simulink subsystem "rail_constraints"  (R2026a)
settings: Solver=VariableStepAuto
undefined symbols (not defined in the file): location, rail_length
settings Model: Creator=finnb  LastModifiedBy=trist

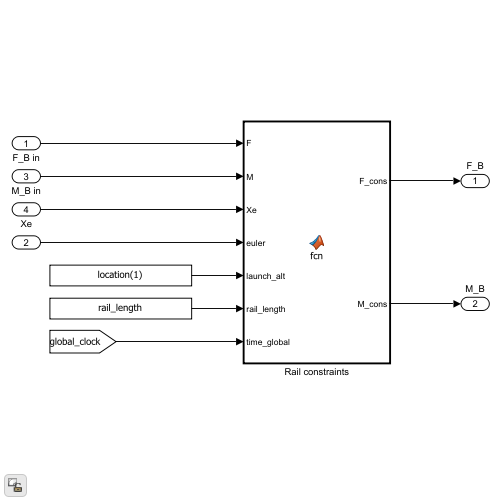
[thumbnail: Simulink's stored preview of the top-level diagram]
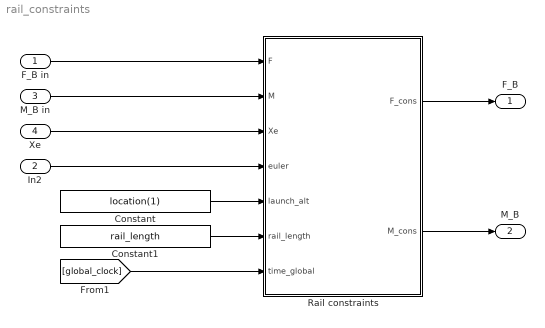
== system rail_constraints ==
  F_B in : Inport
  In2 : Inport  Port=2
  M_B in : Inport  Port=3
  Xe : Inport  Port=4
  Constant : Constant  Value=location(1)
  Constant1 : Constant  Value=rail_length
  Rail constraints : MATLAB Function  TreatAsAtomicUnit=on
  F_B : Outport  VectorParamsAs1DForOutWhenUnconnected=off
  M_B : Outport  Port=2  VectorParamsAs1DForOutWhenUnconnected=off
  wires:
  Xe/1 -> Rail constraints/3(Xe)
  Constant/1 -> Rail constraints/5(launch_alt)
  Rail constraints/1(F_cons) -> F_B/1
  Rail constraints/2(M_cons) -> M_B/1
  F_B in/1 -> Rail constraints/1(F)
  M_B in/1 -> Rail constraints/2(M)
  [global_clock] -> Rail constraints/7(time_global)
  Constant1/1 -> Rail constraints/6(rail_length)
  In2/1 -> Rail constraints/4(euler)

== matlab function rail_constraints/Rail constraints ==
  data: F input; M input; Xe input; euler input; F_cons output; launch_alt input size=1; rail_length input size=1; M_cons output; time_global input
function [F_cons, M_cons] = fcn(F, M, Xe, euler, launch_alt, rail_length, time_global)
    % rail constraints
    
    % not on rail
    F_cons = F;
    M_cons = M;
    
    % before liftoff, on rail
    if time_global <= 0
       F_cons = zeros(3,1);
       M_cons = zeros(3,1);
    
    % after liftoff, on rail
    elseif Xe(1) <= (launch_alt + rail_length)
        % only x direction force on rail
        F_cons = zeros(3,1);
        F_cons(1) = F(1); 
        M_cons = zeros(3,1);

        % no sliding into ground
        if Xe(1) <= launch_alt && F(1) <= 0 % if on stand and net force backwards
            F_cons(1) = 0; % no backwards force 
        end
   end
end
